simulink model "ChiefMaster_TTC580"  (R2022b)
settings: Solver=FixedStepAuto  StartTime=0.0  StopTime=10  FixedStep=0.01  RelTol=1e-3
values from neighbouring files (symbols this model uses):
  BattBox1_No = single(1)    [Parameters.m]
  BattBox2_No = single(2)    [Parameters.m]
  BattBox3_No = single(3)    [Parameters.m]
  CurrentLB = single(-3)    [Parameters.m]
  CurrentReductionConstant_Lvl0 = single(0.03)    [Parameters.m]
  CurrentReductionConstant_Lvl1 = single(0.05)    [Parameters.m]
  CurrentReductionConstant_Lvl2 = single(0.07)    [Parameters.m]
  CurrentReductionConstant_Lvl3 = single(0.1)    [Parameters.m]
  CurrentUB = single(3)    [Parameters.m]
  DCHV_Minus_In_Delay_ms = single(500)    [Parameters.m]
  FL_sHVC_CellBalanceVoltage_mV = single(3500)    [Parameters.m]
  FL_sInrushCurrent_dividebyzero = single(0.00001)    [Parameters.m]
  FL_u8HMI_BuzzerTimer = uint8(3)    [Parameters.m]
  IP_boActValue = true    [Parameters.m]
  IP_boDeactValue = false    [Parameters.m]
  IP_boInitValue = false    [Parameters.m]
  IP_s_LB = 18000    [Parameters.m]
  IP_s_UB = 22000    [Parameters.m]
  IP_sBatt1_ChargeCurrentMax_Factor = single(0.1)    [Parameters.m]
  IP_sBatt1_ChargeCurrentMax_LB = single(0)    [Parameters.m]
  IP_sBatt1_ChargeCurrentMax_Offset = single(0)    [Parameters.m]
  IP_sBatt1_ChargeCurrentMax_UB = single(6553.5)    [Parameters.m]
  IP_sBatt1_Current_Factor = single(0.1)    [Parameters.m]
  IP_sBatt1_Current_LB = single(-3276.8)    [Parameters.m]
  IP_sBatt1_Current_Offset = single(0)    [Parameters.m]
  IP_sBatt1_Current_UB = single(3276.8)    [Parameters.m]
  IP_sBatt1_DisChargeCurrentMax_Factor = single(0.1)    [Parameters.m]
  IP_sBatt1_DisChargeCurrentMax_LB = single(0)    [Parameters.m]
  IP_sBatt1_DisChargeCurrentMax_Offset = single(0)    [Parameters.m]
  IP_sBatt1_DisChargeCurrentMax_UB = single(6553.5)    [Parameters.m]
  IP_sBatt1_InsulationResistance_Factor = single(5)    [Parameters.m]
  IP_sBatt1_InsulationResistance_LB = single(0)    [Parameters.m]
  IP_sBatt1_InsulationResistance_Offset = single(0)    [Parameters.m]
  IP_sBatt1_InsulationResistance_UB = single(0)    [Parameters.m]
  IP_sBatt1_LiBa_IntResist_mOhm = single(25)    [Parameters.m]
  IP_sBatt1_SOC_Factor = single(1)    [Parameters.m]
  IP_sBatt1_SOC_LB = single(0)    [Parameters.m]
  IP_sBatt1_SOC_Offset = single(0)    [Parameters.m]
  IP_sBatt1_SOC_UB = single(100)    [Parameters.m]
  IP_sBatt1_SOH_Factor = single(1)    [Parameters.m]
  IP_sBatt1_SOH_LB = single(0)    [Parameters.m]
  IP_sBatt1_SOH_Offset = single(0)    [Parameters.m]
  IP_sBatt1_SOH_UB = single(100)    [Parameters.m]
  IP_sBatt1_Ubatt_Factor = single(0.1)    [Parameters.m]
  IP_sBatt1_Ubatt_LB = single(0)    [Parameters.m]
  IP_sBatt1_Ubatt_Offset = single(0)    [Parameters.m]
  IP_sBatt1_Ubatt_UB = single(6553.5)    [Parameters.m]
  IP_sBatt1_UserRi_Factor = single(1)    [Parameters.m]
  IP_sBatt1_UserRi_LB = single(0)    [Parameters.m]
  IP_sBatt1_UserRi_Offset = single(0)    [Parameters.m]
  IP_sBatt1_UserRi_UB = single(255)    [Parameters.m]
  IP_sBatt1_VoltageAtSensor_Factor = single(0.02)    [Parameters.m]
  IP_sBatt1_VoltageAtSensor_LB = single(0)    [Parameters.m]
  IP_sBatt1_VoltageAtSensor_Offset = single(0)    [Parameters.m]
  IP_sBatt1_VoltageAtSensor_UB = single(1310.7)    [Parameters.m]
  IP_sBatt2_LiBa_IntResist_mOhm = single(25)    [Parameters.m]
  IP_sBatt3_LiBa_IntResist_mOhm = single(25)    [Parameters.m]
  IP_sEM_LB = 2000    [Parameters.m]
  IP_sEM_UB = 8000    [Parameters.m]
  IP_sFB_LB = 5000    [Parameters.m]
  IP_sFB_UB = 10000    [Parameters.m]
  IP_sHVIL_LB = 12000    [Parameters.m]
  IP_sHVIL_UB = 15000    [Parameters.m]
  IP_sLoad_Voltage_Factor = single(1)    [Parameters.m]
  IP_sLoad_Voltage_LB = single(0)    [Parameters.m]
  IP_sLoad_Voltage_Offset = single(0)    [Parameters.m]
  IP_sLoad_Voltage_UB = single(65535)    [Parameters.m]
  IP_u8HVIL_Delay_ms = uint8(100)    [Parameters.m]
  IP_u8HW_IN_delay_ms = uint8(100)    [Parameters.m]
  IT_sInsulationSafeValue_kOhm = single(650)    [Parameters.m]
  IT_u8IMD_DelayTime_s = uint8(20)    [Parameters.m]
  MainHV_Minus_In_Delay = single(5)    [Parameters.m]
  MainHV_StatusDelay = single(5)    [Parameters.m]
  NotAvailable_uint16 = single(65535)    [Parameters.m]
  NotAvailable_uint8 = uint8(255)    [Parameters.m]
  OP_boHVIL_Supply = boolean(1)    [Parameters.m]
  SafeCurrentToCloseHV_A = single(5)    [Parameters.m]
  SafeVoltageToCloseHV_V = single(0.5)    [Parameters.m]
  UnexpectedBattChargingFcn_Available = boolean(1)    [Parameters.m]
  Voltage_NA_UB = uint16(65535)    [Parameters.m]
  VoltageSensorAvailableBB1 = boolean(0)    [Parameters.m]
  VoltageSensorAvailableBB2 = boolean(0)    [Parameters.m]
  VoltageSensorAvailableBB3 = boolean(0)    [Parameters.m]
libraries: simulink x184, Library_DataProcessing_v1_1 x167, Library_DataProcessing_v1 x142, libCM x28
(part 5 of 19)

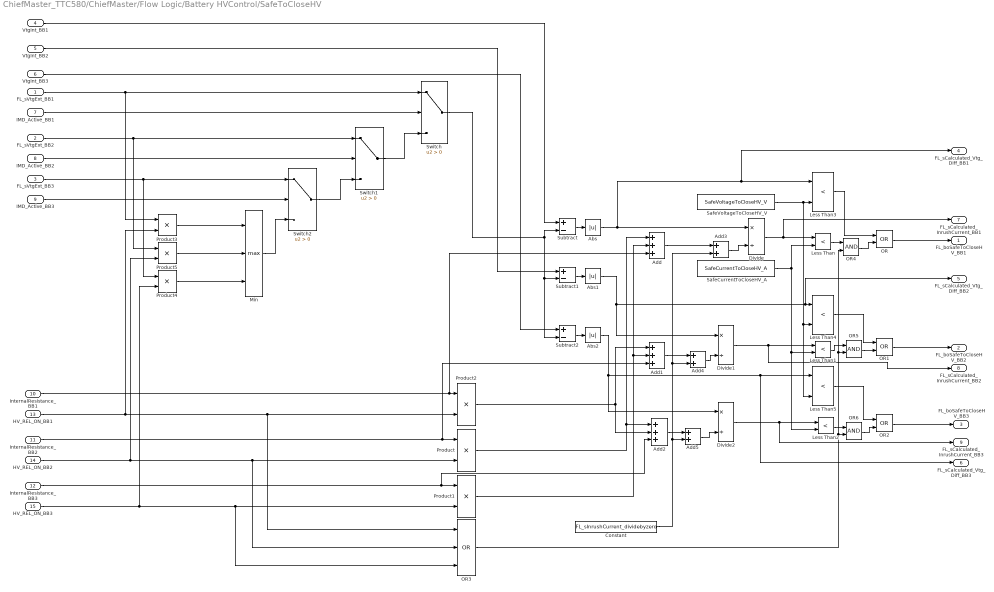
== system ChiefMaster_TTC580/ChiefMaster/Flow Logic/Battery HVControl/SafeToCloseHV ==
  FL_sVtgExt_BB1 : Inport
  FL_sVtgExt_BB2 : Inport  Port=2
  FL_sVtgExt_BB3 : Inport  Port=3
  VtgInt_BB1 : Inport  Port=4
  VtgInt_BB2 : Inport  Port=5
  VtgInt_BB3 : Inport  Port=6
  IMD_Active_BB1 : Inport  Port=7
  IMD_Active_BB2 : Inport  Port=8
  IMD_Active_BB3 : Inport  Port=9
  InternalResistance_BB1 : Inport  Port=10
  InternalResistance_BB2 : Inport  Port=11
  InternalResistance_BB3 : Inport  Port=12
  HV_REL_ON_BB1 : Inport  Port=13
  HV_REL_ON_BB2 : Inport  Port=14
  HV_REL_ON_BB3 : Inport  Port=15
  Abs : Abs  SaturateOnIntegerOverflow=off
  Abs1 : Abs  SaturateOnIntegerOverflow=off
  Abs2 : Abs  SaturateOnIntegerOverflow=off
  Add : Sum  Inputs=+++
  Add1 : Sum  Inputs=+++
  Add2 : Sum  Inputs=+++
  Add3 : Sum
  Add4 : Sum
  Add5 : Sum
  Constant : Constant  Value=FL_sInrushCurrent_dividebyzero  OutDataTypeStr=single
  Divide : Product  Inputs=*/
  Divide1 : Product  Inputs=*/
  Divide2 : Product  Inputs=*/
  Less Than{,1..5} (6 alike) : RelationalOperator  Operator=<  OutDataTypeStr=boolean  RndMeth=Simplest  InputSameDT=off
  Min : MinMax  Function=max  Inputs=3
  OR : Logic  Operator=OR  AllPortsSameDT=off  OutDataTypeStr=boolean
  OR1 : Logic  Operator=OR  AllPortsSameDT=off  OutDataTypeStr=boolean
  OR2 : Logic  Operator=OR  AllPortsSameDT=off  OutDataTypeStr=boolean
  OR3 : Logic  Operator=OR  Inputs=3  AllPortsSameDT=off  OutDataTypeStr=boolean
  OR4 : Logic  AllPortsSameDT=off  OutDataTypeStr=boolean
  OR5 : Logic  AllPortsSameDT=off  OutDataTypeStr=boolean
  OR6 : Logic  AllPortsSameDT=off  OutDataTypeStr=boolean
  Product{,1..5} (6 alike) : Product
  SafeCurrentToCloseHV_A : Constant  Value=SafeCurrentToCloseHV_A
  SafeVoltageToCloseHV_V : Constant  Value=SafeVoltageToCloseHV_V
  Subtract : Sum  Inputs=+-
  Subtract1 : Sum  Inputs=+-
  Subtract2 : Sum  Inputs=+-
  Switch : Switch  Criteria=u2 > Threshold  SaturateOnIntegerOverflow=off  InputSameDT=off
  Switch1 : Switch  Criteria=u2 > Threshold  SaturateOnIntegerOverflow=off  InputSameDT=off
  Switch2 : Switch  Criteria=u2 > Threshold  SaturateOnIntegerOverflow=off  InputSameDT=off
  FL_boSafeToCloseHV_BB1 : Outport
  FL_boSafeToCloseHV_BB2 : Outport  Port=2
  FL_boSafeToCloseHV_BB3 : Outport  Port=3
  FL_sCalculated_Vtg_Diff_BB1 : Outport  Port=4
  FL_sCalculated_Vtg_Diff_BB2 : Outport  Port=5
  FL_sCalculated_Vtg_Diff_BB3 : Outport  Port=6
  FL_sCalculated_InrushCurrent_BB1 : Outport  Port=7
  FL_sCalculated_InrushCurrent_BB2 : Outport  Port=8
  FL_sCalculated_InrushCurrent_BB3 : Outport  Port=9
  wires:
  OR6/1 -> OR2/2
  Less Than1/1 -> OR5/1
  OR5/1 -> OR1/2
  OR4/1 -> OR/2
  OR3/1 -> OR4/2, OR5/2, OR6/2
  Less Than5/1 -> OR2/1
  Less Than4/1 -> OR1/1
  OR2/1 -> FL_boSafeToCloseHV_BB3/1
  OR1/1 -> FL_boSafeToCloseHV_BB2/1
  SafeVoltageToCloseHV_V/1 -> Less Than3/2, Less Than4/2, Less Than5/2
  Less Than3/1 -> OR/1
  OR/1 -> FL_boSafeToCloseHV_BB1/1
  VtgInt_BB3/1 -> Subtract2/1
  VtgInt_BB2/1 -> Subtract1/1
  VtgInt_BB1/1 -> Subtract/1
  Product/1 -> Add2/1, Add/1
  InternalResistance_BB1/1 -> Product2/1, Add/3
  Abs2/1 -> Less Than5/1, FL_sCalculated_Vtg_Diff_BB3/1, Divide2/1
  Abs1/1 -> Divide1/1, Less Than4/1, FL_sCalculated_Vtg_Diff_BB2/1
  Abs/1 -> Divide/1, Less Than3/1, FL_sCalculated_Vtg_Diff_BB1/1
  Switch1/1 -> Switch/3
  FL_sVtgExt_BB3/1 -> Product4/1, Switch2/1
  Switch2/1 -> Switch1/3
  FL_sVtgExt_BB2/1 -> Product5/1, Switch1/1
  FL_sVtgExt_BB1/1 -> Switch/1, Product3/1
  Min/1 -> Switch2/3
  IMD_Active_BB3/1 -> Switch2/2
  SafeCurrentToCloseHV_A/1 -> Less Than/2, Less Than2/2, Less Than1/2
  Less Than2/1 -> OR6/1
  Less Than/1 -> OR4/1
  Divide2/1 -> Less Than2/1, FL_sCalculated_InrushCurrent_BB3/1
  Divide1/1 -> Less Than1/1, FL_sCalculated_InrushCurrent_BB2/1
  Divide/1 -> Less Than/1, FL_sCalculated_InrushCurrent_BB1/1
  Subtract2/1 -> Abs2/1
  Product2/1 -> Add2/2, Add1/1
  IMD_Active_BB1/1 -> Switch/2
  InternalResistance_BB3/1 -> Add2/3, Product1/1
  Product1/1 -> Add1/2, Add/2
  InternalResistance_BB2/1 -> Product/1, Add1/3
  IMD_Active_BB2/1 -> Switch1/2
  Subtract1/1 -> Abs1/1
  Subtract/1 -> Abs/1
  Switch/1 -> Subtract2/2, Subtract1/2, Subtract/2
  Product3/1 -> Min/1
  Product5/1 -> Min/2
  Product4/1 -> Min/3
  Add/1 -> Add3/1
  Add1/1 -> Add4/1
  Add2/1 -> Add5/1
  HV_REL_ON_BB1/1 -> Product3/2, Product2/2, OR3/1
  HV_REL_ON_BB2/1 -> Product5/2, Product/2, OR3/2
  HV_REL_ON_BB3/1 -> Product4/2, Product1/2, OR3/3
  Add3/1 -> Divide/2
  Constant/1 -> Add5/2, Add4/2, Add3/2
  Add4/1 -> Divide1/2
  Add5/1 -> Divide2/2

== system ChiefMaster_TTC580/ChiefMaster/Flow Logic/Battery HVControl/Subsystem ==
  MainHV_Minus_Status : Inport
  MainHV_Plus_Status : Inport  Port=2
  MainHV_WeldingCheckActive : Inport  Port=3
  AND : Logic  Inputs=3  AllPortsSameDT=off  OutDataTypeStr=boolean
  Compare To Constant : simulink/Logic and Bit Operations/Compare To Constant  relop===  const=3  OutDataTypeStr=boolean
  Compare To Constant1 : simulink/Logic and Bit Operations/Compare To Constant  relop===  const=1  OutDataTypeStr=boolean
  Compare To Constant2 : simulink/Logic and Bit Operations/Compare To Constant  relop===  const=3  OutDataTypeStr=boolean
  Compare To Constant3 : simulink/Logic and Bit Operations/Compare To Constant  relop===  const=1  OutDataTypeStr=boolean
  Compare To Constant4 : simulink/Logic and Bit Operations/Compare To Constant  relop===  const=0  OutDataTypeStr=boolean
  NOT : Logic  Operator=NOT  AllPortsSameDT=off  OutDataTypeStr=boolean
  OR : Logic  Operator=OR  AllPortsSameDT=off  OutDataTypeStr=boolean
  OR1 : Logic  Operator=OR  AllPortsSameDT=off  OutDataTypeStr=boolean
  OR2 : Logic  AllPortsSameDT=off  OutDataTypeStr=boolean
  Unit Delay : UnitDelay  SampleTime=-1  HasFrameUpgradeWarning=on
  Unit Delay1 : UnitDelay  SampleTime=-1  HasFrameUpgradeWarning=on
  Unit Delay2 : UnitDelay  SampleTime=-1  HasFrameUpgradeWarning=on
  FL_boMainHV_SD_OK : Outport
  FL_boMainHV_PlusMinus_Status : Outport  Port=2
  wires:
  Compare To Constant/1 -> OR/2
  Compare To Constant1/1 -> OR2/1, OR/1
  Compare To Constant3/1 -> OR2/2, OR1/1
  Compare To Constant2/1 -> OR1/2
  OR/1 -> AND/1
  OR1/1 -> AND/2
  AND/1 -> FL_boMainHV_SD_OK/1
  Unit Delay/1 -> Compare To Constant2/1, Compare To Constant3/1
  Unit Delay1/1 -> Compare To Constant1/1, Compare To Constant/1
  MainHV_Minus_Status/1 -> Unit Delay1/1
  MainHV_Plus_Status/1 -> Unit Delay/1
  MainHV_WeldingCheckActive/1 -> Unit Delay2/1
  Compare To Constant4/1 -> AND/3
  Unit Delay2/1 -> Compare To Constant4/1
  OR2/1 -> NOT/1
  NOT/1 -> FL_boMainHV_PlusMinus_Status/1

== system ChiefMaster_TTC580/ChiefMaster/Flow Logic/Battery HVControl/Voltage_External ==
  VtgInt_BB1 : Inport
  VtgInt_BB2 : Inport  Port=2
  VtgInt_BB3 : Inport  Port=3
  VtgExt_BB1_Sensor : Inport  Port=4
  VtgExt_BB2_Sensor : Inport  Port=5
  VtgExt_BB3_Sensor : Inport  Port=6
  Current_BB1 : Inport  Port=7
  Current_BB2 : Inport  Port=8
  Current_BB3 : Inport  Port=9
  InternalResistance_BB1 : Inport  Port=10
  InternalResistance_BB2 : Inport  Port=11
  InternalResistance_BB3 : Inport  Port=12
  HV_REL_ON_BB1 : Inport  Port=13
  HV_REL_ON_BB2 : Inport  Port=14
  HV_REL_ON_BB3 : Inport  Port=15
  Add : Sum  Inputs=+-
  Add1 : Sum  Inputs=+-
  Add2 : Sum  Inputs=+-
  Constant : Constant  Value=0  OutDataTypeStr=single
  Constant1 : Constant  Value=0  OutDataTypeStr=single
  Constant2 : Constant  Value=0  OutDataTypeStr=single
  Product1 : Product
  Product2 : Product
  Product3 : Product
  Switch{,1..5} (6 alike) : Switch  Criteria=u2 > Threshold  SaturateOnIntegerOverflow=off  InputSameDT=off
  VoltageSensorAvailableBB1 : Constant  Value=VoltageSensorAvailableBB1  OutDataTypeStr=boolean
  VoltageSensorAvailableBB2 : Constant  Value=VoltageSensorAvailableBB2  OutDataTypeStr=boolean
  VoltageSensorAvailableBB3 : Constant  Value=VoltageSensorAvailableBB3  OutDataTypeStr=boolean
  FL_sVtgExt_BB1 : Outport
  FL_sVtgExt_BB2 : Outport  Port=2
  FL_sVtgExt_BB3 : Outport  Port=3
  wires:
  VtgExt_BB1_Sensor/1 -> Switch/1
  InternalResistance_BB1/1 -> Product2/1
  VoltageSensorAvailableBB1/1 -> Switch/2
  VtgInt_BB1/1 -> Add/1
  Product2/1 -> Add/2
  Add/1 -> Switch/3
  Add1/1 -> Switch1/3
  Product3/1 -> Add1/2
  VtgInt_BB2/1 -> Add1/1
  VoltageSensorAvailableBB2/1 -> Switch1/2
  InternalResistance_BB2/1 -> Product3/1
  VtgExt_BB2_Sensor/1 -> Switch1/1
  InternalResistance_BB3/1 -> Product1/1
  VoltageSensorAvailableBB3/1 -> Switch2/2
  VtgInt_BB3/1 -> Add2/1
  Product1/1 -> Add2/2
  Add2/1 -> Switch2/3
  Switch3/1 -> Product2/2
  VtgExt_BB3_Sensor/1 -> Switch2/1
  Switch4/1 -> Product3/2
  Switch5/1 -> Product1/2
  Switch/1 -> FL_sVtgExt_BB1/1
  Switch1/1 -> FL_sVtgExt_BB2/1
  Switch2/1 -> FL_sVtgExt_BB3/1
  Constant2/1 -> Switch5/3
  Current_BB3/1 -> Switch5/1
  HV_REL_ON_BB1/1 -> Switch3/2
  Current_BB1/1 -> Switch3/1
  Current_BB2/1 -> Switch4/1
  HV_REL_ON_BB3/1 -> Switch5/2
  HV_REL_ON_BB2/1 -> Switch4/2
  Constant1/1 -> Switch4/3
  Constant/1 -> Switch3/3

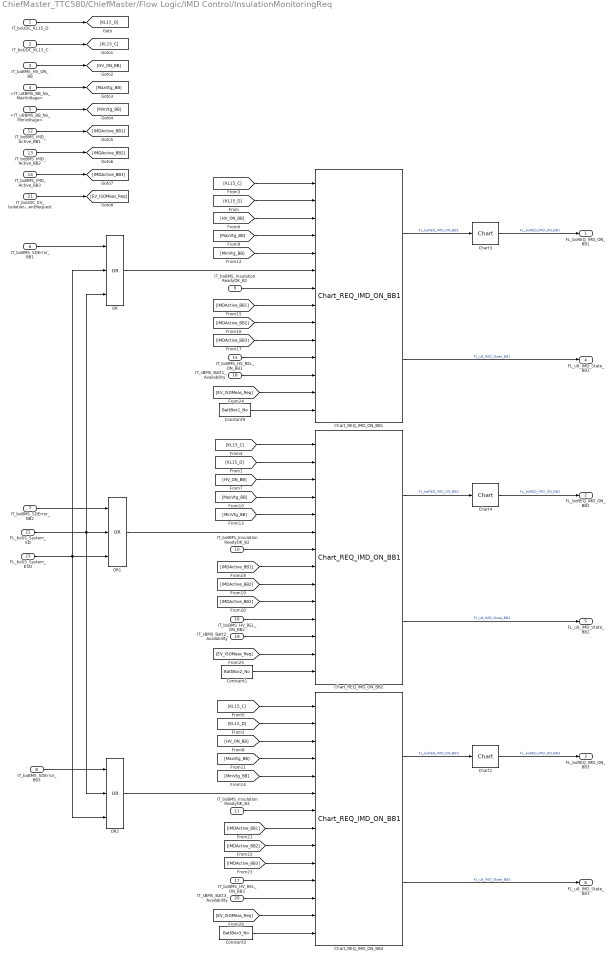
== system ChiefMaster_TTC580/ChiefMaster/Flow Logic/IMD Control/InsulationMonitoringReq ==
  IT_boUDC_KL15_D : Inport
  IT_boUDC_KL15_C : Inport  Port=2
  IT_boBMS_HV_ON_BB : Inport  Port=3
  <IT_u8BMS_BB_No_MaxVoltage> : Inport  Port=4
  <IT_u8BMS_BB_No_MinVoltage> : Inport  Port=5
  IT_boBMS_SDError_BB1 : Inport  Port=6
  IT_boBMS_SDError_BB2 : Inport  Port=7
  IT_boBMS_SDError_BB3 : Inport  Port=8
  IT_boBMS_InsulationReadyOK_B1 : Inport  Port=9
  IT_boBMS_InsulationReadyOK_B2 : Inport  Port=10
  IT_boBMS_InsulationReadyOK_B3 : Inport  Port=11
  IT_boBMS_IMD_Active_BB1 : Inport  Port=12
  IT_boBMS_IMD_Active_BB2 : Inport  Port=13
  IT_boBMS_IMD_Active_BB3 : Inport  Port=14
  IT_boBMS_HV_REL_ON_BB1 : Inport  Port=15
  IT_boBMS_HV_REL_ON_BB2 : Inport  Port=16
  IT_boBMS_HV_REL_ON_BB3 : Inport  Port=17
  IT_sBMS_Batt1_Availability : Inport  Port=18
  IT_sBMS_Batt2_Availability : Inport  Port=19
  IT_sBMS_Batt3_Availability : Inport  Port=20
  IT_boUDC_EV_IsolationMeasurementRequest : Inport  Port=21
  FL_boSS_System_SD : Inport  Port=22
  FL_boSS_System_ESD : Inport  Port=23
  Chart1 : libCM/Chart  SystemSampleTime=-1  VariantActivationTime=update diagram  Latency=0  AutoFrameSizeCalculation=off
  Chart3 : libCM/Chart  SystemSampleTime=-1  VariantActivationTime=update diagram  Latency=0  AutoFrameSizeCalculation=off
  Chart4 : libCM/Chart  SystemSampleTime=-1  VariantActivationTime=update diagram  Latency=0  AutoFrameSizeCalculation=off
  Chart_REQ_IMD_ON_BB1 : libCM/Chart_REQ_IMD_ON_BB1  SystemSampleTime=-1  VariantActivationTime=update diagram  Latency=0  AutoFrameSizeCalculation=off
      settings: PortSchema="{\"entries\":[{\"content\":{\"sides\":[{\"content\":{\"connectorIds\":[\"In1\",\"In2\",\"In8\",\"In4\",\"In5\",\"In6\",\"In3\",\"In11\",\"In9\",\"In10\",\"In12\",\"In13\",\"In14\",\"In7\"]},\"type\":\"ConnectorPlacement.EquallySpacedRectSide\",\"uuid\":\"8d42b6d3-700d-4664-9176-2af1fd91a5ef\"},{\"content\":{\"connectorIds\":[\"Out1\",\"Out2\"],\"side\":\"RIGHT\"},\"type\":\"ConnectorPlacement.EquallySpacedRectSide\",\"uuid\":\"1055ad88-7b4e-4849-9034-0e2b968d970a\"},{\"content\":{\"connectorIds\":[],\"side\":\"TOP\"},\"type\":\"ConnectorPlacement.EquallySpacedRectSide\",\"uuid\":\"93b8508a-130b-4038-9854-7181d979ecdb\"}]},\"type\":\"ConnectorPlacement.EquallySpacedConnector\",\"uuid\":\"712ba1bb-a03e-4078-b3d0-f15207ecb0ed\"}],\"packageUris\":[\"http://schema.mathworks.com/mf0/Connector/R2020b\"],\"version\":\"1.0\"}"
  Chart_REQ_IMD_ON_BB2 : libCM/Chart_REQ_IMD_ON_BB1  SystemSampleTime=-1  VariantActivationTime=update diagram  Latency=0  AutoFrameSizeCalculation=off
      settings: PortSchema="{\"entries\":[{\"content\":{\"sides\":[{\"content\":{\"connectorIds\":[\"In1\",\"In2\",\"In8\",\"In4\",\"In5\",\"In6\",\"In3\",\"In11\",\"In9\",\"In10\",\"In12\",\"In13\",\"In14\",\"In7\"]},\"type\":\"ConnectorPlacement.EquallySpacedRectSide\",\"uuid\":\"8d42b6d3-700d-4664-9176-2af1fd91a5ef\"},{\"content\":{\"connectorIds\":[\"Out1\",\"Out2\"],\"side\":\"RIGHT\"},\"type\":\"ConnectorPlacement.EquallySpacedRectSide\",\"uuid\":\"1055ad88-7b4e-4849-9034-0e2b968d970a\"},{\"content\":{\"connectorIds\":[],\"side\":\"TOP\"},\"type\":\"ConnectorPlacement.EquallySpacedRectSide\",\"uuid\":\"93b8508a-130b-4038-9854-7181d979ecdb\"}]},\"type\":\"ConnectorPlacement.EquallySpacedConnector\",\"uuid\":\"712ba1bb-a03e-4078-b3d0-f15207ecb0ed\"}],\"packageUris\":[\"http://schema.mathworks.com/mf0/Connector/R2020b\"],\"version\":\"1.0\"}"
  Chart_REQ_IMD_ON_BB4 : libCM/Chart_REQ_IMD_ON_BB1  SystemSampleTime=-1  VariantActivationTime=update diagram  Latency=0  AutoFrameSizeCalculation=off
      settings: PortSchema="{\"entries\":[{\"content\":{\"sides\":[{\"content\":{\"connectorIds\":[\"In1\",\"In2\",\"In8\",\"In4\",\"In5\",\"In6\",\"In3\",\"In11\",\"In9\",\"In10\",\"In12\",\"In13\",\"In14\",\"In7\"]},\"type\":\"ConnectorPlacement.EquallySpacedRectSide\",\"uuid\":\"8d42b6d3-700d-4664-9176-2af1fd91a5ef\"},{\"content\":{\"connectorIds\":[\"Out1\",\"Out2\"],\"side\":\"RIGHT\"},\"type\":\"ConnectorPlacement.EquallySpacedRectSide\",\"uuid\":\"1055ad88-7b4e-4849-9034-0e2b968d970a\"},{\"content\":{\"connectorIds\":[],\"side\":\"TOP\"},\"type\":\"ConnectorPlacement.EquallySpacedRectSide\",\"uuid\":\"93b8508a-130b-4038-9854-7181d979ecdb\"}]},\"type\":\"ConnectorPlacement.EquallySpacedConnector\",\"uuid\":\"712ba1bb-a03e-4078-b3d0-f15207ecb0ed\"}],\"packageUris\":[\"http://schema.mathworks.com/mf0/Connector/R2020b\"],\"version\":\"1.0\"}"
  Constant1 : Constant  Value=BattBox2_No
  Constant2 : Constant  Value=BattBox3_No
  Constant9 : Constant  Value=BattBox1_No
  OR : Logic  Operator=OR  Inputs=3  AllPortsSameDT=off  OutDataTypeStr=boolean
  OR1 : Logic  Operator=OR  Inputs=3  AllPortsSameDT=off  OutDataTypeStr=boolean
  OR2 : Logic  Operator=OR  Inputs=3  AllPortsSameDT=off  OutDataTypeStr=boolean
  FL_boREQ_IMD_ON_BB1 : Outport  OutDataTypeStr=boolean
  FL_boREQ_IMD_ON_BB2 : Outport  Port=2  OutDataTypeStr=boolean
  FL_boREQ_IMD_ON_BB3 : Outport  Port=3  OutDataTypeStr=boolean
  FL_u8_IMD_State_BB1 : Outport  Port=4  OutDataTypeStr=uint8
  FL_u8_IMD_State_BB2 : Outport  Port=5  OutDataTypeStr=uint8
  FL_u8_IMD_State_BB3 : Outport  Port=6  OutDataTypeStr=uint8
  wires:
  Constant9/1 -> Chart_REQ_IMD_ON_BB1/7
  IT_boBMS_InsulationReadyOK_B1/1 -> Chart_REQ_IMD_ON_BB1/3
  IT_boUDC_KL15_C/1 -> [KL15_C]
  IT_boUDC_KL15_D/1 -> [KL15_D]
  OR/1 -> Chart_REQ_IMD_ON_BB1/6
  Chart_REQ_IMD_ON_BB1/1 -> Chart3/1  "FL_boREQ_IMD_ON_BB1"
  Constant2/1 -> Chart_REQ_IMD_ON_BB4/7
  IT_boBMS_InsulationReadyOK_B3/1 -> Chart_REQ_IMD_ON_BB4/3
  OR2/1 -> Chart_REQ_IMD_ON_BB4/6
  IT_boBMS_HV_ON_BB/1 -> [HV_ON_BB]
  OR1/1 -> Chart_REQ_IMD_ON_BB2/6
  IT_boBMS_InsulationReadyOK_B2/1 -> Chart_REQ_IMD_ON_BB2/3
  IT_boBMS_HV_REL_ON_BB1/1 -> Chart_REQ_IMD_ON_BB1/12
  IT_boBMS_HV_REL_ON_BB2/1 -> Chart_REQ_IMD_ON_BB2/12
  IT_boBMS_HV_REL_ON_BB3/1 -> Chart_REQ_IMD_ON_BB4/12
  IT_boBMS_SDError_BB1/1 -> OR/1
  FL_boSS_System_SD/1 -> OR/3, OR2/2, OR1/2
  FL_boSS_System_ESD/1 -> OR1/3, OR2/3, OR/2
  IT_boBMS_SDError_BB2/1 -> OR1/1
  IT_boBMS_SDError_BB3/1 -> OR2/1
  Chart_REQ_IMD_ON_BB2/1 -> Chart4/1  "FL_boREQ_IMD_ON_BB2"
  Chart_REQ_IMD_ON_BB4/1 -> Chart1/1  "FL_boREQ_IMD_ON_BB3"
  IT_sBMS_Batt3_Availability/1 -> Chart_REQ_IMD_ON_BB4/13
  IT_sBMS_Batt1_Availability/1 -> Chart_REQ_IMD_ON_BB1/13
  IT_sBMS_Batt2_Availability/1 -> Chart_REQ_IMD_ON_BB2/13
  [KL15_D] -> Chart_REQ_IMD_ON_BB1/2
  [KL15_D] -> Chart_REQ_IMD_ON_BB2/2
  [KL15_D] -> Chart_REQ_IMD_ON_BB4/2
  [KL15_C] -> Chart_REQ_IMD_ON_BB1/1
  [KL15_C] -> Chart_REQ_IMD_ON_BB2/1
  [KL15_C] -> Chart_REQ_IMD_ON_BB4/1
  [HV_ON_BB] -> Chart_REQ_IMD_ON_BB1/8
  [HV_ON_BB] -> Chart_REQ_IMD_ON_BB2/8
  [HV_ON_BB] -> Chart_REQ_IMD_ON_BB4/8
  <IT_u8BMS_BB_No_MaxVoltage>/1 -> [MaxVtg_BB]
  [MaxVtg_BB] -> Chart_REQ_IMD_ON_BB1/4
  [MaxVtg_BB] -> Chart_REQ_IMD_ON_BB2/4
  [MaxVtg_BB] -> Chart_REQ_IMD_ON_BB4/4
  <IT_u8BMS_BB_No_MinVoltage>/1 -> [MinVtg_BB]
  [MinVtg_BB] -> Chart_REQ_IMD_ON_BB1/5
  [MinVtg_BB] -> Chart_REQ_IMD_ON_BB2/5
  [MinVtg_BB] -> Chart_REQ_IMD_ON_BB4/5
  IT_boBMS_IMD_Active_BB1/1 -> [IMDActive_BB1]
  IT_boBMS_IMD_Active_BB2/1 -> [IMDActive_BB2]
  IT_boBMS_IMD_Active_BB3/1 -> [IMDActive_BB3]
  [IMDActive_BB1] -> Chart_REQ_IMD_ON_BB1/11
  [IMDActive_BB2] -> Chart_REQ_IMD_ON_BB1/9
  [IMDActive_BB3] -> Chart_REQ_IMD_ON_BB1/10
  [IMDActive_BB1] -> Chart_REQ_IMD_ON_BB2/11
  [IMDActive_BB2] -> Chart_REQ_IMD_ON_BB2/9
  [IMDActive_BB3] -> Chart_REQ_IMD_ON_BB2/10
  [IMDActive_BB1] -> Chart_REQ_IMD_ON_BB4/11
  [IMDActive_BB2] -> Chart_REQ_IMD_ON_BB4/9
  [IMDActive_BB3] -> Chart_REQ_IMD_ON_BB4/10
  Constant1/1 -> Chart_REQ_IMD_ON_BB2/7
  IT_boUDC_EV_IsolationMeasurementRequest/1 -> [EV_ISOMeas_Req]
  [EV_ISOMeas_Req] -> Chart_REQ_IMD_ON_BB1/14
  [EV_ISOMeas_Req] -> Chart_REQ_IMD_ON_BB2/14
  [EV_ISOMeas_Req] -> Chart_REQ_IMD_ON_BB4/14
  Chart3/1 -> FL_boREQ_IMD_ON_BB1/1  "FL_boREQ_IMD_ON_BB1"
  Chart4/1 -> FL_boREQ_IMD_ON_BB2/1  "FL_boREQ_IMD_ON_BB2"
  Chart1/1 -> FL_boREQ_IMD_ON_BB3/1  "FL_boREQ_IMD_ON_BB3"
  Chart_REQ_IMD_ON_BB1/2 -> FL_u8_IMD_State_BB1/1  "FL_u8_IMD_State_BB1"
  Chart_REQ_IMD_ON_BB2/2 -> FL_u8_IMD_State_BB2/1  "FL_u8_IMD_State_BB2"
  Chart_REQ_IMD_ON_BB4/2 -> FL_u8_IMD_State_BB3/1  "FL_u8_IMD_State_BB3"

== system ChiefMaster_TTC580/ChiefMaster/Flow Logic/KL15/System_KL15 ==
  IT_boHW_KL15 : Inport
  IT_boUDC_KL15_D : Inport  Port=2
  IT_boUDC_KL15_C : Inport  Port=3
  Reset_BB1 : Inport  Port=4
  Reset_BB2 : Inport  Port=5
  Reset_BB3 : Inport  Port=6
  Contactor_FB_State_BB1 : Inport  Port=7
  Contactor_FB_State_BB2 : Inport  Port=8
  Contactor_FB_State_BB3 : Inport  Port=9
  AND : Logic  Inputs=4  AllPortsSameDT=off  OutDataTypeStr=boolean
  AND6 : Logic  Operator=NXOR  AllPortsSameDT=off  OutDataTypeStr=boolean
  NOR : Logic  Operator=NOR  Inputs=3  AllPortsSameDT=off  OutDataTypeStr=boolean
  NOT{1..4} (4 alike) : Logic  Operator=NOT  AllPortsSameDT=off  OutDataTypeStr=boolean
  Subsystem : libCM/Subsystem  SystemSampleTime=-1  VariantActivationTime=update diagram  Latency=0  AutoFrameSizeCalculation=off
  Subsystem1 : libCM/Subsystem  SystemSampleTime=-1  VariantActivationTime=update diagram  Latency=0  AutoFrameSizeCalculation=off
  Subsystem3 : libCM/Subsystem  SystemSampleTime=-1  VariantActivationTime=update diagram  Latency=0  AutoFrameSizeCalculation=off
  FL_boCMSleep : Outport
  FL_boKL15_BB1 : Outport  Port=2
  FL_boKL15_BB2 : Outport  Port=3
  FL_boKL15_BB3 : Outport  Port=4
  FL_boKL15_Disable : Outport  Port=5
  FL_boKL15_Reset : Outport  Port=6
  wires:
  IT_boHW_KL15/1 -> Subsystem3/1, NOT1/1, Subsystem1/1, Subsystem/1, NOR/3
  Subsystem3/1 -> NOT2/1, FL_boKL15_BB1/1  "FL_boKL15_BB1"
  Subsystem/1 -> NOT4/1, FL_boKL15_BB3/1  "FL_boKL15_BB3"
  Reset_BB1/1 -> Subsystem3/2
  Reset_BB2/1 -> Subsystem1/2
  Reset_BB3/1 -> Subsystem/2
  Contactor_FB_State_BB1/1 -> Subsystem3/3
  Contactor_FB_State_BB2/1 -> Subsystem1/3
  Contactor_FB_State_BB3/1 -> Subsystem/3
  AND6/1 -> FL_boKL15_Disable/1  "FL_boKL15_Disable"
  NOR/1 -> FL_boKL15_Reset/1  "FL_boKL15_Reset"
  Subsystem1/1 -> NOT3/1, FL_boKL15_BB2/1  "FL_boKL15_BB2"
  AND/1 -> FL_boCMSleep/1  "FL_boCMSleep"
  NOT1/1 -> AND/1
  NOT2/1 -> AND/2
  NOT3/1 -> AND/3
  NOT4/1 -> AND/4
  IT_boUDC_KL15_D/1 -> NOR/1, AND6/1
  IT_boUDC_KL15_C/1 -> NOR/2, AND6/2

== system ChiefMaster_TTC580/ChiefMaster/Flow Logic/Reset/Reset_Req ==
  KL_15_BB1 : Inport
  KL_15_BB2 : Inport  Port=2
  KL_15_BB3 : Inport  Port=3
  ChargeMode : Inport  Port=4
  DriveMode : Inport  Port=5
  MaxVtgBB : Inport  Port=6
  MinVtgBB : Inport  Port=7
  SDError_BB1 : Inport  Port=8
  SDError_BB2 : Inport  Port=9
  SDError_BB3 : Inport  Port=10
  ContactorState_BB1 : Inport  Port=11
  ContactorState_BB2 : Inport  Port=12
  ContactorState_BB3 : Inport  Port=13
  Compare To Constant : simulink/Logic and Bit Operations/Compare To Constant  relop===  const=1  OutDataTypeStr=boolean
  Compare To Constant1 : simulink/Logic and Bit Operations/Compare To Constant  relop===  const=1  OutDataTypeStr=boolean
  Compare To Constant2 : simulink/Logic and Bit Operations/Compare To Constant  relop===  const=2  OutDataTypeStr=boolean
  Compare To Constant3 : simulink/Logic and Bit Operations/Compare To Constant  relop===  const=2  OutDataTypeStr=boolean
  Compare To Constant4 : simulink/Logic and Bit Operations/Compare To Constant  relop===  const=3  OutDataTypeStr=boolean
  Compare To Constant5 : simulink/Logic and Bit Operations/Compare To Constant  relop===  const=3  OutDataTypeStr=boolean
  Constant : Constant  Value=3
  OR : Logic  Operator=OR  Inputs=3  AllPortsSameDT=off  OutDataTypeStr=boolean
  OR1 : Logic  Operator=OR  Inputs=3  AllPortsSameDT=off  OutDataTypeStr=boolean
  OR2 : Logic  Operator=OR  AllPortsSameDT=off  OutDataTypeStr=boolean
  OR3 : Logic  Operator=OR  AllPortsSameDT=off  OutDataTypeStr=boolean
  OR4 : Logic  Operator=OR  AllPortsSameDT=off  OutDataTypeStr=boolean
  Subsystem1 : libCM/Subsystem6  SystemSampleTime=-1  VariantActivationTime=update diagram  Latency=0  AutoFrameSizeCalculation=off
  Subsystem2 : libCM/Subsystem6  SystemSampleTime=-1  VariantActivationTime=update diagram  Latency=0  AutoFrameSizeCalculation=off
  Subsystem3 : libCM/Subsystem3  SystemSampleTime=-1  VariantActivationTime=update diagram  Latency=0  AutoFrameSizeCalculation=off
  Subsystem4 : libCM/Subsystem3  SystemSampleTime=-1  VariantActivationTime=update diagram  Latency=0  AutoFrameSizeCalculation=off
  Subsystem5 : libCM/Subsystem3  SystemSampleTime=-1  VariantActivationTime=update diagram  Latency=0  AutoFrameSizeCalculation=off
  Subsystem7 : libCM/Subsystem6  SystemSampleTime=-1  VariantActivationTime=update diagram  Latency=0  AutoFrameSizeCalculation=off
  Software_Reset_KL15_BB1 : Outport
  Software_Reset_KL15_BB2 : Outport  Port=2
  Software_Reset_KL15_BB3 : Outport  Port=3
  Manual_Reset_KL15_ALL : Outport  Port=4
  Software_Reset_KL15_ALL : Outport  Port=5
  wires:
  OR/1 -> OR2/2, OR3/2, OR4/2, Software_Reset_KL15_ALL/1  "Software_Reset_KL15_ALL"
  OR1/1 -> Manual_Reset_KL15_ALL/1  "Manual_Reset_KL15_ALL"
  ChargeMode/1 -> Subsystem7/1, Subsystem2/1, Subsystem1/1, Subsystem5/3, Subsystem4/3, Subsystem3/3
  MaxVtgBB/1 -> Compare To Constant5/1, Compare To Constant2/1, Compare To Constant/1
  MinVtgBB/1 -> Compare To Constant4/1, Compare To Constant3/1, Compare To Constant1/1
  ContactorState_BB1/1 -> Subsystem7/4
  Compare To Constant/1 -> Subsystem7/2
  Compare To Constant1/1 -> Subsystem7/3
  Subsystem7/1 -> OR/1
  Subsystem7/2 -> OR1/1
  Subsystem1/1 -> OR/2
  Subsystem1/2 -> OR1/2
  Subsystem2/1 -> OR/3
  Subsystem2/2 -> OR1/3
  Compare To Constant3/1 -> Subsystem1/3
  Compare To Constant2/1 -> Subsystem1/2
  Compare To Constant5/1 -> Subsystem2/2
  Compare To Constant4/1 -> Subsystem2/3
  ContactorState_BB2/1 -> Subsystem1/4
  ContactorState_BB3/1 -> Subsystem2/4
  SDError_BB3/1 -> Subsystem5/1
  SDError_BB2/1 -> Subsystem4/1
  SDError_BB1/1 -> Subsystem3/1
  Constant/1 -> Subsystem3/5, Subsystem5/5, Subsystem4/5
  OR2/1 -> Software_Reset_KL15_BB1/1  "Software_Reset_KL15_BB1"
  OR3/1 -> Software_Reset_KL15_BB2/1  "Software_Reset_KL15_BB2"
  OR4/1 -> Software_Reset_KL15_BB3/1  "Software_Reset_KL15_BB3"
  DriveMode/1 -> Subsystem3/4, Subsystem5/4, Subsystem4/4
  KL_15_BB1/1 -> Subsystem3/2
  KL_15_BB2/1 -> Subsystem4/2
  KL_15_BB3/1 -> Subsystem5/2
  Subsystem5/1 -> OR4/1  "Software_Reset_KL15_ALL"
  Subsystem4/1 -> OR3/1
  Subsystem3/1 -> OR2/1

== system ChiefMaster_TTC580/ChiefMaster/Flow Logic/System Status/AlarmBuzzer ==
  SSD : Inport
  ESD : Inport  Port=2
  Chart : Stateflow chart  TreatAsAtomicUnit=on
  Constant : Constant  OutDataTypeStr=boolean
  Constant1 : Constant  Value=0  OutDataTypeStr=boolean
  Constant2 : Constant  Value=FL_u8HMI_BuzzerTimer  OutDataTypeStr=uint8
  OR3 : Logic  Operator=OR  Inputs=3  AllPortsSameDT=off  OutDataTypeStr=boolean
  Switch : Switch  Criteria=u2 > Threshold  SaturateOnIntegerOverflow=off  InputSameDT=off
  FL_boSS_CabinAlarm : Outport
  wires:
  OR3/1 -> Switch/2
  Constant2/1 -> Chart/1(BuzzerTimer)
  Constant/1 -> Switch/1
  ESD/1 -> OR3/2  "ESD"
  Chart/1(out) -> OR3/3
  Constant1/1 -> Switch/3
  Switch/1 -> FL_boSS_CabinAlarm/1  "FL_boSS_CabinAlarm"
  SSD/1 -> OR3/1  "SSD"

== system ChiefMaster_TTC580/ChiefMaster/Flow Logic/System Status/CMState ==
  KL15 : Inport
  KL15_AllBoxes : Inport  Port=2
  InsulationReadyOK : Inport  Port=3
  BattRelay_Closed : Inport  Port=4
  IMD_Available : Inport  Port=5
  BattRelay_Close_Req : Inport  Port=6
  REQ_IMD_ON : Inport  Port=7
  FL_boREQ_MainHV_ON_MINUS : Inport  Port=8
  MainHV_Plus_Status : Inport  Port=9
  ShutdownError : Inport  Port=10
  CMState : Stateflow chart  TreatAsAtomicUnit=on
      settings: PortSchema="{\"entries\":[{\"content\":{\"sides\":[{\"content\":{\"connectorIds\":[\"In1\",\"In3\",\"In10\",\"In6\",\"In7\",\"In8\",\"In2\",\"In4\",\"In5\",\"In9\"]},\"type\":\"ConnectorPlacement.EquallySpacedRectSide\",\"uuid\":\"0898174c-83fe-48f3-a774-7848044d39bf\"},{\"content\":{\"connectorIds\":[\"Out1\"],\"side\":\"RIGHT\"},\"type\":\"ConnectorPlacement.EquallySpacedRectSide\",\"uuid\":\"488d7238-f562-4096-bb02-81587daf3494\"},{\"content\":{\"connectorIds\":[],\"side\":\"TOP\"},\"type\":\"ConnectorPlacement.EquallySpacedRectSide\",\"uuid\":\"6eae4935-dd59-41d2-8a16-60d5218dfe9b\"}]},\"type\":\"ConnectorPlacement.EquallySpacedConnector\",\"uuid\":\"9700ce03-6ddb-408b-85b3-8fdeb5603cae\"}],\"packageUris\":[\"http://schema.mathworks.com/mf0/Connector/R2020b\"],\"version\":\"1.0\"}"
  FL_u8SS_ChiefMaster_State : Outport  OutDataTypeStr=uint8
  wires:
  IMD_Available/1 -> CMState/10(IMD_Available)
  FL_boREQ_MainHV_ON_MINUS/1 -> CMState/2(FL_boREQ_MainHV_ON_MINUS)
  BattRelay_Close_Req/1 -> CMState/7(BattRelay_Close_Req)
  ShutdownError/1 -> CMState/9(ShutdownError)
  InsulationReadyOK/1 -> CMState/6(InsulationReadyOK)
  KL15_AllBoxes/1 -> CMState/3(KL15_AllBoxes)
  CMState/1(CMState) -> FL_u8SS_ChiefMaster_State/1  "FL_u8SS_ChiefMaster_State"
  REQ_IMD_ON/1 -> CMState/8(REQ_IMD_ON)
  KL15/1 -> CMState/1(KL15)
  MainHV_Plus_Status/1 -> CMState/5(MainHV_Plus_Status)
  BattRelay_Closed/1 -> CMState/4(BattRelay_Closed)

== system ChiefMaster_TTC580/ChiefMaster/Flow Logic/System Status/CurrentPrognosis ==
  FL_boST_System_Error : Inport
  FL_boST_System_SD : Inport  Port=2
  FL_boST_System_ESD : Inport  Port=3
  IT_Databus : Inport  Port=4
  FL_boKL15_Disable : Inport  Port=5
  FL_boSS_BDU_Reset : Inport  Port=6
  FL_u8SS_NumberOfConnectedBatt : Inport  Port=7
  AND : Logic  Inputs=3  AllPortsSameDT=off  OutDataTypeStr=boolean
  Add : Sum  Inputs=+++
  BattChargeFcn : Stateflow chart  TreatAsAtomicUnit=on
      settings: RTWSystemCode=Reusable function  RTWFcnNameOpts=Use subsystem name  RTWFileNameOpts=Use subsystem name  PortSchema="{\"entries\":[{\"content\":{\"sides\":[{\"content\":{\"connectorIds\":[\"In1\",\"In2\",\"In3\",\"In4\",\"In5\",\"In6\",\"In7\",\"In8\",\"In9\",\"In10\",\"In11\",\"In12\"]},\"type\":\"ConnectorPlacement.EquallySpacedRectSide\",\"uuid\":\"21cff15b-7665-4626-94ff-475fd60be04f\"},{\"content\":{\"connectorIds\":[\"Out1\",\"Out4\",\"Out2\",\"Out3\",\"Out5\"],\"side\":\"RIGHT\"},\"type\":\"ConnectorPlacement.EquallySpacedRectSide\",\"uuid\":\"b21296f4-23de-4bce-9305-41ec0860bdab\"},{\"content\":{\"connectorIds\":[],\"side\":\"TOP\"},\"type\":\"ConnectorPlacement.EquallySpacedRectSide\",\"uuid\":\"40e28fde-017d-46be-a22d-9d553271eb10\"}]},\"type\":\"ConnectorPlacement.EquallySpacedConnector\",\"uuid\":\"efd3b07c-da6d-47b7-909f-f85c812edbed\"}],\"packageUris\":[\"http://schema.mathworks.com/mf0/Connector/R2020b\"],\"version\":\"1.0\"}"
  Bus Selector : BusSelector  OutputSignals=IT_BatterySignal_Databus.IT_sBMS_ChargeCurrentPrognosis_BB1,IT_BatterySignal_Databus.IT_sBMS_ChargeCurrentPrognosis_BB2,IT_BatterySignal_Databus.IT_sBMS_ChargeCurrentPrognosis_BB3,IT_BatterySignal_Databus.IT_boBMS_HV_REL_ON_BB1,IT_BatterySignal_Databus.IT_boBMS_HV_REL_ON_BB2,IT_BatterySignal_Databus.IT_boBMS_HV_REL_ON_BB3,IT_BatterySignal_Databus.IT_sBMS_DisChargeCurrentPrognosis_BB1,IT_BatterySignal_Databus.IT_sBMS_DisChargeCurrentPrognosis_BB2,IT_BatterySignal_Databus.IT_sBMS_DisChargeCurrentPrognosis_BB3
  Bus Selector1 : BusSelector  OutputSignals=IT_UDC_Databus.IT_boChargeStop_Button,IT_BatterySignal_Databus.IT_boBMS_HV_REL_ON_BB1,IT_BatterySignal_Databus.IT_boBMS_HV_REL_ON_BB2,IT_BatterySignal_Databus.IT_boBMS_HV_REL_ON_BB3,IT_BatterySignal_Databus.IT_sBMS_Current_BB1,IT_BatterySignal_Databus.IT_sBMS_Current_BB2,IT_BatterySignal_Databus.IT_sBMS_Current_BB3
  Compare To Constant : simulink/Logic and Bit Operations/Compare To Constant  relop=>  const=1  OutDataTypeStr=boolean
  Compare To Constant1 : simulink/Logic and Bit Operations/Compare To Constant  relop===  const=0  OutDataTypeStr=boolean
  Constant : Constant  Value=UnexpectedBattChargingFcn_Available
  Constant1 : Constant  Value=NotAvailable_uint16  OutDataTypeStr=single
  Constant2 : Constant  Value=0  OutDataTypeStr=single
  Constant3 : Constant  Value=UnexpectedBattChargingFcn_Available
  Constant4 : Constant  Value=0
  Constant5 : Constant  Commented=on  Value=CurrentLB
  Constant6 : Constant  Value=CurrentUB
  Min : MinMax  Inputs=3
  Min1 : MinMax  Inputs=3
  NOR1 : Logic  Operator=OR  Inputs=3  AllPortsSameDT=off  OutDataTypeStr=boolean
  NOT : Logic  Operator=NOT  AllPortsSameDT=off  OutDataTypeStr=boolean
  OR : Logic  Operator=OR  Inputs=3  AllPortsSameDT=off  OutDataTypeStr=boolean
  OR2 : Logic  Operator=OR  Inputs=3  AllPortsSameDT=off  OutDataTypeStr=boolean
  Product1 : Product  Inputs=3
  Product2 : Product  Inputs=3
  Subsystem : Subsystem
  Switch{,1..7} (8 alike) : Switch  Criteria=u2 > Threshold  SaturateOnIntegerOverflow=off  InputSameDT=off
  Unit Delay : UnitDelay  InitialCondition=1  SampleTime=-1  HasFrameUpgradeWarning=on
  FL_sSS_MaxChargeCurrent : Outport
  FL_sSS_MaxDisChargeCurrent : Outport  Port=2
  FL_boST_REQ_HV_Open_Batt1 : Outport  Port=3
  FL_boSS_REQ_HV_Open_Batt2 : Outport  Port=4
  FL_boSS_REQ_HV_Open_Batt3 : Outport  Port=5
  FL_boST_BatteryReadyToShutDown : Outport  Port=6
  wires:
  Switch2/1 -> Min/3
  Switch/1 -> Min/1
  Bus Selector/1 -> Switch/1  "<IT_sBMS_ChargeCurrentPrognosis_BB1>"
  Min/1 -> Product2/1
  Switch1/1 -> Min/2
  Bus Selector/2 -> Switch1/1  "<IT_sBMS_ChargeCurrentPrognosis_BB2>"
  Bus Selector/3 -> Switch2/1  "<IT_sBMS_ChargeCurrentPrognosis_BB3>"
  Bus Selector/5 -> Switch1/2, OR/2, Switch5/2, Add/2  "<IT_boBMS_HV_REL_ON_BB2>"
  Switch3/1 -> Switch6/3, Switch5/3, Switch4/3, Switch/3, Switch1/3, Switch2/3
  Bus Selector/6 -> Switch6/2, Add/3, Switch2/2, OR/3  "<IT_boBMS_HV_REL_ON_BB3>"
  Add/1 -> Product1/1, Product2/2
  OR/1 -> Switch3/2
  Constant1/1 -> Switch3/1
  Constant2/1 -> Switch3/3
  Switch5/1 -> Min1/2
  Min1/1 -> Product1/2
  Switch4/1 -> Min1/1
  Bus Selector/8 -> Switch5/1  "<IT_sBMS_DisChargeCurrentPrognosis_BB2>"
  Switch6/1 -> Min1/3
  Bus Selector/7 -> Switch4/1  "<IT_sBMS_DisChargeCurrentPrognosis_BB1>"
  Product1/1 -> FL_sSS_MaxDisChargeCurrent/1  "FL_sSS_MaxDisChargeCurrent"
  Bus Selector/9 -> Switch6/1  "<IT_sBMS_DisChargeCurrentPrognosis_BB3>"
  Bus Selector/4 -> Switch4/2, Add/1, OR/1, Switch/2  "<IT_boBMS_HV_REL_ON_BB1>"
  OR2/1 -> NOT/1
  NOT/1 -> Product2/3, Product1/3
  FL_boST_System_Error/1 -> NOR1/3
  FL_boST_System_SD/1 -> NOR1/2
  FL_boST_System_ESD/1 -> NOR1/1
  NOR1/1 -> OR2/2
  FL_boSS_BDU_Reset/1 -> OR2/1
  Constant4/1 -> Switch7/1
  Bus Selector1/4 -> Subsystem/3(<IP_boBMS_HV_REL_ON_BB3>), BattChargeFcn/6(HV_ON_Batt3)  "<IT_boBMS_HV_REL_ON_BB3>"
  Switch7/1 -> OR2/3
  Constant3/1 -> Switch7/2
  Constant/1 -> AND/1
  Bus Selector1/2 -> Subsystem/1(<IP_boBMS_HV_REL_ON_BB1>), BattChargeFcn/4(HV_ON_Batt1)  "<IT_boBMS_HV_REL_ON_BB1>"
  Bus Selector1/5 -> Subsystem/4(<IP_sBMS_Current_BB1>), BattChargeFcn/7(Ibatt1)  "<IT_sBMS_Current_BB1>"
  IT_Databus/1 -> Bus Selector/1, Bus Selector1/1
  Constant6/1 -> BattChargeFcn/12(CurrentUB)
  Product2/1 -> BattChargeFcn/2(MaxChargeCurrentBatt)
  FL_boKL15_Disable/1 -> Switch7/3, Compare To Constant1/1
  BattChargeFcn/1(FL_sST_MaxChargeCurrent) -> FL_sSS_MaxChargeCurrent/1, Unit Delay/1  "FL_sSS_MaxChargeCurrent"
  BattChargeFcn/5(BatteryReadyToShutDown) -> FL_boST_BatteryReadyToShutDown/1  "FL_boSS_BatteryReadyToShutDown"
  Subsystem/1(CurrentReductionConstant) -> BattChargeFcn/11(CurrentReductionConstant)
  Compare To Constant/1 -> AND/2
  Compare To Constant1/1 -> AND/3
  Constant5/1 -> ?
  FL_u8SS_NumberOfConnectedBatt/1 -> Compare To Constant/1
  BattChargeFcn/2(REQ_HV_Open_Batt2) -> FL_boSS_REQ_HV_Open_Batt2/1  "FL_boSS_REQ_HV_Open_Batt2"
  BattChargeFcn/4(REQ_HV_Open_Batt1) -> FL_boST_REQ_HV_Open_Batt1/1  "FL_boSS_REQ_HV_Open_Batt1"
  Bus Selector1/3 -> Subsystem/2(<IP_boBMS_HV_REL_ON_BB2>), BattChargeFcn/5(HV_ON_Batt2)  "<IT_boBMS_HV_REL_ON_BB2>"
  AND/1 -> BattChargeFcn/10(Fcn_available)
  BattChargeFcn/3(REQ_HV_Open_Batt3) -> FL_boSS_REQ_HV_Open_Batt3/1  "FL_boSS_REQ_HV_Open_Batt3"
  Unit Delay/1 -> BattChargeFcn/1(MaxChargeCurr_fb)
  Bus Selector1/6 -> Subsystem/5(<IP_sBMS_Current_BB2>), BattChargeFcn/8(Ibatt2)  "<IT_sBMS_Current_BB2>"
  Bus Selector1/7 -> Subsystem/6(<IP_sBMS_Current_BB3>), BattChargeFcn/9(Ibatt3)  "<IT_sBMS_Current_BB3>"
  Bus Selector1/1 -> BattChargeFcn/3(ChargeStopPressed)  "<IT_boChargeStop_Button>"

== system ChiefMaster_TTC580/ChiefMaster/Flow Logic/System Status/EMSRET_Power ==
  ESD : Inport
  HVILNOK : Inport  Port=2
  Reset : Inport  Port=3
  AND : Logic  AllPortsSameDT=off  OutDataTypeStr=boolean
  EMSRET : Stateflow chart  TreatAsAtomicUnit=on
      settings: RTWSystemCode=Reusable function  RTWFcnNameOpts=Use subsystem name  RTWFileNameOpts=Use subsystem name
  NOT : Logic  Operator=NOT  AllPortsSameDT=off  OutDataTypeStr=boolean
  NOT1 : Logic  Operator=NOT  AllPortsSameDT=off  OutDataTypeStr=boolean
  FL_boSS_EMSRET_POWER : Outport
  wires:
  NOT1/1 -> AND/1
  NOT/1 -> AND/2
  HVILNOK/1 -> NOT/1
  AND/1 -> EMSRET/1(AllOK)  "FL_boSS_EMSRET_POWER"
  ESD/1 -> NOT1/1
  Reset/1 -> EMSRET/2(Reset)
  EMSRET/1(EMSRET) -> FL_boSS_EMSRET_POWER/1  "FL_boSS_EMSRET_POWER"

== system ChiefMaster_TTC580/ChiefMaster/Flow Logic/System Status/EmergencySD ==
  FL_boKL15_Reset : Inport
  <IT_boEmergencySwitch_NC> : Inport  Port=2
  <IT_boEmergencySwitch_NO> : Inport  Port=3
  <IT_boHW_HVIL_BDU> : Inport  Port=4
  <IT_boHW_HVIL_Components> : Inport  Port=5
  <IT_boHW_HVIL_Battery> : Inport  Port=6
  <IT_boHW_HVIL_Overrule> : Inport  Port=7
  IT_boHW_ResetButton_LED_NO_State : Inport  Port=8
  AND : Logic  AllPortsSameDT=off  OutDataTypeStr=boolean
  Compare To Constant : simulink/Logic and Bit Operations/Compare To Constant  relop=>=  const=1  OutDataTypeStr=boolean
  Constant : Constant  Value=0  OutDataTypeStr=boolean
  Emergency_Switch_Control : Subsystem
  HVIL_NOK : Subsystem  TreatAsAtomicUnit=on
      settings: RTWFcnNameOpts=Use subsystem name  RTWFileNameOpts=Use subsystem name
  NOT : Logic  Operator=NOT  AllPortsSameDT=off  OutDataTypeStr=boolean
  OR1 : Logic  Operator=OR  AllPortsSameDT=off  OutDataTypeStr=boolean
  Switch : Switch  Criteria=u2 > Threshold  SaturateOnIntegerOverflow=off  InputSameDT=off
  FL_boSS_System_ESD : Outport
  FL_u8SS_EmergencyStopState : Outport  Port=2
  FL_boHVIL_NOK : Outport  Port=3
  wires:
  OR1/1 -> FL_boSS_System_ESD/1  "FL_boSS_System_ESD"
  <IT_boEmergencySwitch_NC>/1 -> Emergency_Switch_Control/2(IT_boEmergencySwitch_NC_S2)
  <IT_boEmergencySwitch_NO>/1 -> Emergency_Switch_Control/3(IT_boVS_EmergencySwitch_NO_S1)
  Emergency_Switch_Control/1(FL_u8VS_EmergencyStopState) -> FL_u8SS_EmergencyStopState/1, Compare To Constant/1  "FL_u8SS_EmergencyStopState"
  <IT_boHW_HVIL_Overrule>/1 -> Switch/2
  Switch/1 -> OR1/2, FL_boHVIL_NOK/1  "FL_boSS_HVIL_NOK"
  Compare To Constant/1 -> OR1/1
  Constant/1 -> Switch/1
  FL_boKL15_Reset/1 -> NOT/1
  IT_boHW_ResetButton_LED_NO_State/1 -> AND/1
  NOT/1 -> AND/2
  AND/1 -> HVIL_NOK/1(boReset), Emergency_Switch_Control/1(reset)
  <IT_boHW_HVIL_BDU>/1 -> HVIL_NOK/2(<IT_boHW_HVIL_BDU>)
  <IT_boHW_HVIL_Components>/1 -> HVIL_NOK/3(<IT_boHW_HVIL_Components>)
  <IT_boHW_HVIL_Battery>/1 -> HVIL_NOK/4(<IT_boHW_HVIL_Battery>)
  HVIL_NOK/1(FL_boSS_HVIL_NOK) -> Switch/3

== system ChiefMaster_TTC580/ChiefMaster/Flow Logic/System Status/Reset_LEDButton ==
  ESD : Inport
  <IT_boHW_ResetButton_LED_NO> : Inport  Port=2
  Constant1 : Constant  Value=false  OutDataTypeStr=boolean
  Constant3 : Constant  Value=false  OutDataTypeStr=boolean
  Constant6 : Constant  Value=true  OutDataTypeStr=boolean
  Data Type Conversion30 : DataTypeConversion  OutDataTypeStr=boolean  SaturateOnIntegerOverflow=off  RndMeth=Floor
  Discrete Pulse Generator20 : DiscretePulseGenerator  Period=100  PulseWidth=50  SampleTime=0.01
  Switch : Switch  Criteria=u2 > Threshold  SaturateOnIntegerOverflow=off  InputSameDT=off
  Switch1 : Switch  Criteria=u2 > Threshold  SaturateOnIntegerOverflow=off  InputSameDT=off
  Switch2 : Switch  Criteria=u2 > Threshold  SaturateOnIntegerOverflow=off  InputSameDT=off
  FL_boSS_ResetButton_LED : Outport
  wires:
  Data Type Conversion30/1 -> Switch/1
  Switch1/1 -> FL_boSS_ResetButton_LED/1  "FL_boSS_ResetButton_LED"
  Discrete Pulse Generator20/1 -> Data Type Conversion30/1
  Constant1/1 -> Switch/3
  Switch/1 -> Switch1/3
  Switch2/1 -> Switch1/1
  Constant6/1 -> Switch2/1
  Constant3/1 -> Switch2/3
  ESD/1 -> Switch/2
  <IT_boHW_ResetButton_LED_NO>/1 -> Switch1/2, Switch2/2

== system ChiefMaster_TTC580/ChiefMaster/Flow Logic/System Status/SDError ==
  FL_boKL15_Reset : Inport
  IT_Databus : Inport  Port=2
  FL_BDUControl_Databus : Inport  Port=3
  FL_BatteryBox_HVControl_Databus : Inport  Port=4
  FL_u8SS_EmergencySD : Inport  Port=5
  Add : Sum  Inputs=+++++++++
  BDU_Error : Subsystem  TreatAsAtomicUnit=on
      settings: RTWFcnNameOpts=Use subsystem name  RTWFileNameOpts=Use subsystem name
  Bus Selector : BusSelector  OutputSignals=IT_BatterySignal_Databus.IT_boBMS_SDError_BB1,IT_BatterySignal_Databus.IT_boBMS_HV_REL_ON_BB1,IT_BatterySignal_Databus.IT_boBMS_SDError_BB2,IT_BatterySignal_Databus.IT_boBMS_HV_REL_ON_BB2,IT_BatterySignal_Databus.IT_boBMS_SDError_BB3,IT_BatterySignal_Databus.IT_boBMS_HV_REL_ON_BB3,IT_BatterySignal_Databus.IT_u8BMS_No_of_Battery_Usable
  Chart : Stateflow chart  TreatAsAtomicUnit=on
      settings: PortSchema="{\"entries\":[{\"content\":{\"sides\":[{\"content\":{\"connectorIds\":[\"In2\",\"In1\"]},\"type\":\"ConnectorPlacement.EquallySpacedRectSide\",\"uuid\":\"4468c933-87b9-48ff-b369-68617597cd7e\"},{\"content\":{\"connectorIds\":[\"Out1\"],\"side\":\"RIGHT\"},\"type\":\"ConnectorPlacement.EquallySpacedRectSide\",\"uuid\":\"d393ad52-ef42-4ebd-906e-4c040c8b1e43\"},{\"content\":{\"connectorIds\":[],\"side\":\"TOP\"},\"type\":\"ConnectorPlacement.EquallySpacedRectSide\",\"uuid\":\"7aa8d615-5bd1-49d2-bf04-a344c9a1c6d2\"}]},\"type\":\"ConnectorPlacement.EquallySpacedConnector\",\"uuid\":\"04e47330-e4e0-4b55-96d2-317153c7b2c3\"}],\"packageUris\":[\"http://schema.mathworks.com/mf0/Connector/R2020b\"],\"version\":\"1.0\"}"
  Compare To Constant : simulink/Logic and Bit Operations/Compare To Constant  relop===  const=0  OutDataTypeStr=boolean
  Constant : Constant  Value=0  OutDataTypeStr=boolean
  Gain : Gain
  Gain1 : Gain  Gain=2
  Gain2 : Gain  Gain=4
  Gain3 : Gain  Gain=8
  Gain4 : Gain  Gain=16
  Gain5 : Gain  Gain=32
  Gain6 : Gain  Gain=64
  Gain7 : Gain  Gain=128
  Gain8 : Gain  Gain=255
  IMD_Error : Subsystem  TreatAsAtomicUnit=on
      settings: RTWFcnNameOpts=Use subsystem name  RTWFileNameOpts=Use subsystem name
  IMD_SD : Subsystem  TreatAsAtomicUnit=on
      settings: RTWFcnNameOpts=Use subsystem name  RTWFileNameOpts=Use subsystem name
  OR : Logic  Operator=OR  Inputs=9  AllPortsSameDT=off  OutDataTypeStr=boolean
  Subsystem : Subsystem
  Subsystem1 : libCM/Subsystem5  SystemSampleTime=-1  VariantActivationTime=update diagram  Latency=0  AutoFrameSizeCalculation=off
  Subsystem2 : libCM/Subsystem5  SystemSampleTime=-1  VariantActivationTime=update diagram  Latency=0  AutoFrameSizeCalculation=off
  Subsystem3 : libCM/Subsystem5  SystemSampleTime=-1  VariantActivationTime=update diagram  Latency=0  AutoFrameSizeCalculation=off
  Subsystem6 : Subsystem
  Terminator : Terminator
  FL_boSS_System_SD : Outport
  FL_u8SS_System_SD_ErrorCode : Outport  Port=2
  wires:
  IMD_SD/1(IMD_SDError) -> Terminator/1, Gain6/1  "IMD_SDError"
  Gain6/1 -> Add/7
  Subsystem6/1(SecuritySwitchError) -> Gain7/1, OR/8  "SecuritySwitchError"
  Bus Selector/2 -> Subsystem1/2  "<IT_boBMS_HV_REL_ON_BB1>"
  Bus Selector/1 -> Subsystem1/1  "<IT_boBMS_SDError_BB1>"
  Subsystem1/1 -> Gain/1, OR/1  "FL_boBatt1_SDError"
  Bus Selector/4 -> Subsystem2/2  "<IT_boBMS_HV_REL_ON_BB2>"
  Bus Selector/3 -> Subsystem2/1  "<IT_boBMS_SDError_BB2>"
  Subsystem2/1 -> Gain1/1, OR/2  "FL_boBatt2_SDError"
  Bus Selector/6 -> Subsystem3/2  "<IT_boBMS_HV_REL_ON_BB3>"
  Bus Selector/5 -> Subsystem3/1  "<IT_boBMS_SDError_BB3>"
  Subsystem3/1 -> Gain2/1, OR/3  "FL_boBatt3_SDError"
  FL_BDUControl_Databus/1 -> BDU_Error/1(Main_REL_Databus)
  BDU_Error/1(BDU_Error) -> Gain3/1, OR/4  "BDU_Error"
  Compare To Constant/1 -> Subsystem3/3, Subsystem2/3, Subsystem1/3
  Bus Selector/7 -> Compare To Constant/1  "<IT_u8BMS_No_of_Battery_Usable>"
  Add/1 -> FL_u8SS_System_SD_ErrorCode/1  "System_SD_ErrorCode"
  Gain5/1 -> Add/6
  Gain4/1 -> Add/5
  Gain3/1 -> Add/4
  Gain2/1 -> Add/3
  Gain1/1 -> Add/2
  Gain/1 -> Add/1
  IMD_Error/1(IMD_Error) -> Gain5/1, OR/6  "IMD_Error"
  FL_BatteryBox_HVControl_Databus/1 -> Subsystem/2(BattPack_REL_Databus)
  IT_Databus/1 -> Subsystem6/1(BatteryPackSignals), IMD_SD/1(BatteryPackSignals), IMD_Error/1(BatteryPackSignals), Subsystem/3(BatteryPackSignals), Bus Selector/1
  Chart/1(System_Error) -> FL_boSS_System_SD/1
  Subsystem/1(REL_Error_BB) -> Gain4/1, OR/5  "REL_Error_BB"
  FL_boKL15_Reset/1 -> Subsystem/1(KL15_Reset), Chart/2(KL15_CM_reset)
  OR/1 -> Chart/1(In)
  Gain7/1 -> Add/8
  FL_u8SS_EmergencySD/1 -> Gain8/1, OR/9  "FL_u8SS_EmergencySD"
  Gain8/1 -> Add/9
  Constant/1 -> OR/7

== system ChiefMaster_TTC580/ChiefMaster/Flow Logic/System Status/SafetoSD ==
  FL_boST_BatteryReadyToShutDown : Inport
  <IP_sBMS_Current_BB1> : Inport  Port=2
  <IP_sBMS_Current_BB2> : Inport  Port=3
  <IP_sBMS_Current_BB3> : Inport  Port=4
  <IP_boCM_SafeToSD> : Inport  Port=5
  AND : Logic  Inputs=4  AllPortsSameDT=off  OutDataTypeStr=boolean
  AND1 : Logic  Operator=OR  AllPortsSameDT=off  OutDataTypeStr=boolean
  AND2 : Logic  AllPortsSameDT=off  OutDataTypeStr=boolean
  Abs : Abs  SaturateOnIntegerOverflow=off
  Abs1 : Abs  SaturateOnIntegerOverflow=off
  Abs2 : Abs  SaturateOnIntegerOverflow=off
  Compare To Constant1 : simulink/Logic and Bit Operations/Compare To Constant  relop=<=  const=1  OutDataTypeStr=boolean
  Compare To Constant2 : simulink/Logic and Bit Operations/Compare To Constant  relop=<=  const=1  OutDataTypeStr=boolean
  Compare To Constant3 : simulink/Logic and Bit Operations/Compare To Constant  relop=<=  const=1  OutDataTypeStr=boolean
  Constant : Constant  Value=UnexpectedBattChargingFcn_Available
  Switch : Switch  Criteria=u2 > Threshold  SaturateOnIntegerOverflow=off  InputSameDT=off
  FL_boSS_SafeToSD : Outport
  wires:
  FL_boST_BatteryReadyToShutDown/1 -> AND2/2
  AND1/1 -> Switch/1
  AND2/1 -> AND1/2
  <IP_sBMS_Current_BB2>/1 -> Abs1/1
  Switch/1 -> FL_boSS_SafeToSD/1  "FL_boSS_SafeToSD"
  <IP_sBMS_Current_BB3>/1 -> Abs2/1
  <IP_sBMS_Current_BB1>/1 -> Abs/1
  Abs1/1 -> Compare To Constant2/1
  Compare To Constant1/1 -> AND/1
  Abs/1 -> Compare To Constant1/1
  AND/1 -> AND1/1
  <IP_boCM_SafeToSD>/1 -> Switch/3, AND/4, AND2/1
  Compare To Constant3/1 -> AND/3
  Abs2/1 -> Compare To Constant3/1
  Compare To Constant2/1 -> AND/2
  Constant/1 -> Switch/2
